simulink model "vehicle_motion_model_final_temp"  (R2021b)
settings: Solver=ode5  StartTime=0.0  StopTime=600  FixedStep=0.001  RelTol=1e-3
StopFcn:
  | % stop simulation callback function
  | figure(1);
  | out.x_gt.data = permute(out.x_gt.data,[3, 1, 2]);
  | plot3(out.x_gt.data(:, 1), out.x_gt.data(:, 2), -out.x_gt.data(:, 3), 'Color', 'r', 'LineWidth', 1.5);
  | legend('Истинная траектория')
  | xlabel('X, \itм');
  | ylabel('Y, \itм');
  | zlabel('Z, \itм');
  | figure(2);
  | plot3(out.x.data(:, 1), out.x.data(:, 2), -out.x.data(:, 3), 'Color', 'b', 'LineWidth', 1.5);
  | hold on;
  | xlabel('X, \itм');
  | ylabel('Y, \itм');
  | zlabel('Z, \itм');
  | % legend('pos')
  | hold on;
  | plot3(out.x_gt.data(:, 1), out.x_gt.data(:, 2), -out.x_gt.data(:, 3), 'Color', 'r', 'LineWidth', 1.5);
  | hold on;
  | legend('Рассчитанная траектория', 'Истинная траектория')
  | % errors
  | figure(3);
  | yyaxis left;
  | plot(out.hor_err_fus.time, out.hor_err_fus.data, 'Color', 'b', 'LineWidth', 1.5);
  | xlabel('время, \itс');
  | ylabel('Горизонтальная ошибка, \itм');
  | hold on;
  | yyaxis right;
  | plot(out.ver_err_fus.time, out.ver_err_fus.data, 'Color', 'r', 'LineWidth', 1.5);
  | ylabel('Вертикальная ошибка, \itм');
  | legend('Горизонтальная позиционная ошибка', 'Вертикальная позиционная ошибка');
  | grid on;
  | figure(4);
  | yyaxis left;
  | plot(out.hor_err_ins.time, out.hor_err_ins.data, '-', 'Color', 'b', 'LineWidth', 1.5);
  | xlabel('время, \itс');
  | ylabel('Горизонтальная ошибка, \itм');
  | hold on;
  | yyaxis right;
  | plot(out.ver_err_ins.time, out.ver_err_ins.data, '-', 'Color', 'r', 'LineWidth', 1.5);
  | ylabel('Вертикальная ошибка, \itм');
  | legend('Горизонтальная позиционная ошибка', 'Вертикальная позиционная ошибка');
  | grid on;
model workspace (MAT data in the model file):
  AxlIxx = 62.3745166667
  AxlM = 160
  Cps = 2
  CzWhlAxl = 557955.087061
  DCT_Param : object (value not decoded)
  Downshift_Speeds = [9.5625 12.9375 16.3125 19.6875 23.0625 26.4375 29.8125 33.1875 36.5625 39.9375 43.3125 46.6875 ... (28 elements, 4x7)]
  F0zWhlAxl = 16132.2380068
  HTCH : object (value not decoded)
  Hmax = 0.25
  KzWhlAxl = 58428920.0848
  NCyl = 6
  Pedal_Positions = [0.1 0.4 0.5 0.9]
  Pstd = 101325
  Q = [1  0  0; 0  1  0; 0  0  1]
  Rair = 287
  SUS : object (value not decoded)
  TRA : object (value not decoded)
  Trans : object (value not decoded)
  Tstd = 293.15
  Upshift_Speeds = [12.9375 16.3125 19.6875 33 26.4375 29.8125 33.1875 52.5 39.9375 43.3125 46.6875 77.25 ... (28 elements, 4x7)]
  VEH : object (value not decoded)
  Vd = 0.00346
  WH : Mass (value not decoded)
  dt3D = 0.05
  f_air = [0 0 0 0 0 0 0 0 0 0 0 0 ... (256 elements, 16x16)]
  f_co = [0 0 0 0 0 0 0 0 0 0 0 0 ... (256 elements, 16x16)]
  f_co2 = [0 0 0 0 0 0 0 0 0 0 0 0 ... (256 elements, 16x16)]
  f_eff = [352.135682859 352.135682859 320.724378192 303.655312657 295.930136708 291.240087194 291.240271258 291.240312459 291.240275452 291.240198499 291.240100781 291.240018769 ... (256 elements, 16x16)]
  f_fuel = [0 0 0 0 0 0 0 0 0 0 0 0 ... (256 elements, 16x16)]
  f_hc = [0 0 0 0 0 0 0 0 0 0 0 0 ... (256 elements, 16x16)]
  f_nox = [0 0 0 0 0 0 0 0 0 0 0 0 ... (256 elements, 16x16)]
  f_pm = [0 0 0 0 0 0 0 0 0 0 0 0 ... (256 elements, 16x16)]
  f_susp_axl_bp = [1 2]
  f_susp_dz_bp = [-0.325022776267 -0.315022776267 -0.305022776267 -0.205022776267 -0.105022776267 -0.00502277626717 0.0949772237328 0.194977223733 0.204977223733 0.214977223733]
  f_susp_dzdot_bp = [-3 -0.3 -0.2 -0.1 0 0.1 0.2 0.3 3]
  f_susp_fmz = [-144070.391448 -93629.24037 -75929.1118915 -20630.5828179 -15385.48216 -10140.3815021 -4895.28084414 349.819813785 -31916.3973792 18437.6709544 -83996.1993354 -33555.0482577 ... (43920 elements, 10x9x61x2x4)]
  f_susp_geom = [0 0 0 0 0 0 0 0 0 0 0 0 ... (3660 elements, 10x61x2x3)]
  f_susp_strgdelta_bp = [-0.523598775598 -0.506145483078 -0.488692190558 -0.471238898038 -0.453785605519 -0.436332312999 -0.418879020479 -0.401425727959 -0.383972435439 -0.366519142919 -0.349065850399 -0.331612557879 ... (61 elements, 1x61)]
  f_tbrake = [0 76.8593923996 105.140482948 131.533638111 157.926793274 176.658631717 176.65727296 176.656856686 176.656879077 176.657093756 176.657404516 176.65772406 ... (256 elements, 16x16)]
  f_tbrake_n_bpt = [0 649.519052838 912.419621844 1175.32019085 1438.22075986 1701.12132886 1964.02189787 2226.92246687 2489.82303588 2752.72360489 3015.62417389 3278.5247429 ... (16 elements, 1x16)]
  f_tbrake_t_bpt = [0 34.6410161514 61.0341713143 87.4273264773 113.82048164 140.213636803 166.606791966 192.999947129 219.393102292 245.786257455 272.179412618 298.572567781 ... (16 elements, 1x16)]
  f_texh = [766.752464599 766.752464599 786.17542386 801.679939032 884.591982581 910.574397722 910.571871054 910.570774534 910.570601632 910.570821151 910.571247242 910.571639815 ... (256 elements, 16x16)]
  f_twc_eff_co = [0.17 0.25 0.45 0.99 0.99 0.99 0.99]
  f_twc_eff_hc = [0.21 0.375 0.75 0.98 0.98 0.98 0.98]
  f_twc_eff_lam = [0.909090909 0.944055944 0.979020979 1 1.013986014 1.048951049 1.083916084]
  f_twc_eff_nox = [0.98 0.98 0.98 0.97 0.05 0.02 0]
  h = 0.134
symbols that are objects in the model workspace (value not decoded): VEH
libraries: aerolibcommonsys x8, sharedtransform x8, sharedutil x7, autolibsharedcommon x7, autolibutils x4, vehdynlibtirecommon x3, dspstat3 x2, mspsensorlib x1, aerolibnav x1, shared6dof x1, autolibshared x1, vehdynlibsuspension x1
(part 3 of 9)

== system vehicle_motion_model_final_temp/BINS/Three-axis Inertial Measurement Unit4 ==
  A_b : Inport  Unit=m/s^2  PortDimensions=3
  w : Inport  Port=2  Unit=rad/s  PortDimensions=3
  w_dot : Inport  Port=3  Unit=rad/s^2  PortDimensions=3
  CG : Inport  Port=4  Unit=m  PortDimensions=3
  g : Inport  Port=5  Unit=m/s^2  PortDimensions=3
  Acceleration Conversion : Subsystem
  Disallow CGS : UnitConfiguration  UnitSystemsStr=English,SI,SI (extended)  AllowAllUnitSystems=off
  Three-axis Accelerometer : Subsystem  AncestorBlock=aerolibnav/Three-axis Accelerometer  mask(Three-axis Accelerometer){units=Metric (MKS), acc=imu, gtype=on, dtype_a=off, w_a=w_a, z_a=z_a, a_sf_cc=a_sf_cc, a_bias=a_bias, a_Ts=i_Ts, a_rand=on, a_seeds=i_seeds(1:3), a_pow=i_pow(1:3), a_sat=a_sat}
      mask prompts: units "aeroblks:aeroblknav:blockThreeaxisAccelerometerParamUnits"; acc "aeroblks:aeroblknav:blockThreeaxisAccelerometerParamAccelerometerlocation"; gtype "aeroblks:aeroblknav:blockThreeaxisAccelerometerParamSubtractgravity"; dtype_a "aeroblks:aeroblknav:blockThreeaxisAccelerometerParamSecondorderdynamics"; w_a "aeroblks:aeroblknav:blockThreeaxisAccelerometerParamNaturalfrequencyradsec"; z_a "aeroblks:aeroblknav:blockThreeaxisAccelerometerParamDampingratio"; a_sf_cc "aeroblks:aeroblknav:blockThreeaxisAccelerometerParamScalefactorsandcrosscoupling"; a_bias "aeroblks:aeroblknav:blockThreeaxisAccelerometerParamMeasurementbias"; a_Ts "aeroblks:aeroblknav:blockThreeaxisAccelerometerParamUpdateratesec"; a_rand "aeroblks:aeroblknav:blockThreeaxisAccelerometerParamNoiseon"; a_seeds "aeroblks:aeroblknav:blockThreeaxisAccelerometerParamNoiseseeds"; a_pow "aeroblks:aeroblknav:blockThreeaxisAccelerometerParamNoisepower"; a_sat "aeroblks:aeroblknav:blockThreeaxisAccelerometerParamLowerandupperoutputlimits"
      mask help: aeroblks:aeroblknav:blockThreeaxisAccelerometerDesc
      mask init:
      | par = a_Ts;
      | block = gcb;
      | ports=aeroicon('aeroblkaccel','icon',par);
      | a_satl = a_sat(1:3);
      | a_sath = a_sat(4:6);
      mask Help: eval('asbhelp');
      mask TypeOptions units: aeroblks:aeroblknav:blockThreeaxisAccelerometerParamComboMetricMKS | aeroblks:aeroblknav:blockThreeaxisAccelerometerParamComboEnglish
      mask Callback gtype: aeroicon('aeroblkaccel')
      mask Callback dtype_a: aeroicon('aeroblkaccel')
      mask Callback a_rand: aeroicon('aeroblkaccel')
      mask DialogControl ParameterTabVar0 Prompt: Main
      mask DialogControl units Prompt: Units:
      mask DialogControl acc Prompt: Accelerometer location:
      mask DialogControl gtype Prompt: Subtract gravity:
      mask DialogControl dtype_a Prompt: Second-order dynamics
      mask DialogControl w_a Prompt: Natural frequency (rad/sec):
      mask DialogControl z_a Prompt: Damping ratio:
      mask DialogControl a_sf_cc Prompt: Scale factors and cross-coupling:
      mask DialogControl a_bias Prompt: Measurement bias:
      mask DialogControl a_Ts Prompt: Update rate (sec):
      mask DialogControl ParameterTabVar01 Prompt: Noise
      mask DialogControl a_rand Prompt: Noise on
      mask DialogControl a_seeds Prompt: Noise seeds:
      mask DialogControl a_pow Prompt: Noise power:
      mask DialogControl a_sat Prompt: Lower and upper output limits:
      mask Display:
      | port_label(ports(1).type,ports(1).port,ports(1).txt,'texmode','on');
      | port_label(ports(2).type,ports(2).port,ports(2).txt,'texmode','on');
      | port_label(ports(3).type,ports(3).port,ports(3).txt,'texmode','on');
      | port_label(ports(4).type,ports(4).port,ports(4).txt,'texmode','on');
      | port_label(ports(5).type,ports(5).port,ports(5).txt,'texmode','on');
      | port_label(ports(6).type,ports(6).port,ports(6).txt,'texmode','on');
  Three-axis Gyroscope : Subsystem  AncestorBlock=aerolibnav/Three-axis Gyroscope  mask(Three-axis Gyroscope){dtype_g=off, w_g=w_g, z_g=z_g, g_sf_cc=g_sf_cc, g_bias=g_bias, g_sen=g_sens, g_Ts=i_Ts, g_rand=on, g_seeds=i_seeds(4:6), g_pow=i_pow(4:6), g_sat=g_sat}
      mask prompts: dtype_g "aeroblks:aeroblknav:blockThreeaxisGyroscopeParamSecondorderdynamics"; w_g "aeroblks:aeroblknav:blockThreeaxisGyroscopeParamNaturalfrequencyradsec"; z_g "aeroblks:aeroblknav:blockThreeaxisGyroscopeParamDampingratio"; g_sf_cc "aeroblks:aeroblknav:blockThreeaxisGyroscopeParamScalefactorsandcrosscoupling"; g_bias "aeroblks:aeroblknav:blockThreeaxisGyroscopeParamMeasurementbias"; g_sen "aeroblks:aeroblknav:blockThreeaxisGyroscopeParamGsensitivebias"; g_Ts "aeroblks:aeroblknav:blockThreeaxisGyroscopeParamUpdateratesec"; g_rand "aeroblks:aeroblknav:blockThreeaxisGyroscopeParamNoiseon"; g_seeds "aeroblks:aeroblknav:blockThreeaxisGyroscopeParamNoiseseeds"; g_pow "aeroblks:aeroblknav:blockThreeaxisGyroscopeParamNoisepower"; g_sat "aeroblks:aeroblknav:blockThreeaxisGyroscopeParamLowerandupperoutputlimits"
      mask help: aeroblks:aeroblknav:blockThreeaxisGyroscopeDesc
      mask init:
      | par = g_Ts;
      | block = gcb;
      | g_satl = g_sat(1:3);
      | g_sath = g_sat(4:6);
      | ports=aeroicon('aeroblkgyro','icon',par);
      mask Help: eval('asbhelp');
      mask Callback dtype_g: aeroicon('aeroblkgyro');
      mask Callback g_rand: aeroicon('aeroblkgyro');
      mask DialogControl ParameterTabVar0 Prompt: Main
      mask DialogControl dtype_g Prompt: Second-order dynamics
      mask DialogControl w_g Prompt: Natural frequency (rad/sec):
      mask DialogControl z_g Prompt: Damping ratio:
      mask DialogControl g_sf_cc Prompt: Scale factors and cross-coupling:
      mask DialogControl g_bias Prompt: Measurement bias:
      mask DialogControl g_sen Prompt: G-sensitive bias:
      mask DialogControl g_Ts Prompt: Update rate (sec):
      mask DialogControl ParameterTabVar01 Prompt: Noise
      mask DialogControl g_rand Prompt: Noise on
      mask DialogControl g_seeds Prompt: Noise seeds:
      mask DialogControl g_pow Prompt: Noise power:
      mask DialogControl g_sat Prompt: Lower and upper output limits:
      mask Display:
      | port_label(ports(1).type,ports(1).port,ports(1).txt,'texmode','on');
      | port_label(ports(2).type,ports(2).port,ports(2).txt,'texmode','on');
      | port_label(ports(3).type,ports(3).port,ports(3).txt,'texmode','on');
  A_meas : Outport  Unit=m/s^2  VectorParamsAs1DForOutWhenUnconnected=off
  w_meas : Outport  Port=2  Unit=rad/s  VectorParamsAs1DForOutWhenUnconnected=off
  wires:
  g/1 -> Three-axis Accelerometer/5(g)
  Acceleration Conversion/1(inherit) -> Three-axis Gyroscope/2(G's)
  w_dot/1 -> Three-axis Accelerometer/3(pdot qdot rdot)
  CG/1 -> Three-axis Accelerometer/4(CG)
  w/1 -> Three-axis Accelerometer/2(p q r), Three-axis Gyroscope/1(p q r)
  A_b/1 -> Three-axis Accelerometer/1(Ab), Acceleration Conversion/1(acceleration)
  Three-axis Gyroscope/1((p q r)_meas) -> w_meas/1
  Three-axis Accelerometer/1(Ameas) -> A_meas/1

== system vehicle_motion_model_final_temp/BINS kinematics Euler/Subsystem ==
  True : Inport
  BINS : Inport  Port=2
  Scope1 : Scope  NumInputPorts=3
  Sum2 : Sum  Inputs=+-|
  wires:
  True/1 -> Sum2/1, Scope1/1
  BINS/1 -> Scope1/2, Sum2/2
  Sum2/1 -> Scope1/3

== system vehicle_motion_model_final_temp/BINS kinematics Euler/Subsystem1 ==
  True : Inport
  BINS : Inport  Port=2
  Scope1 : Scope  NumInputPorts=3
  Sum2 : Sum  Inputs=+-|
  wires:
  True/1 -> Sum2/1, Scope1/1
  BINS/1 -> Scope1/2, Sum2/2
  Sum2/1 -> Scope1/3

== system vehicle_motion_model_final_temp/Calc errors/Subsystem ==
  <Disp> : Inport
  <CalcPos> : Inport  Port=2
  Abs : Abs
  Selector : Selector  InputPortWidth=3  IndexOptions=Index vector (dialog)  Indices=[1]  OutputSizes=1
  Selector1 : Selector  InputPortWidth=3  IndexOptions=Index vector (dialog)  Indices=[1]  OutputSizes=1
  Selector2 : Selector  InputPortWidth=3  IndexOptions=Index vector (dialog)  Indices=[2]  OutputSizes=1
  Selector3 : Selector  InputPortWidth=3  IndexOptions=Index vector (dialog)  Indices=[2]  OutputSizes=1
  Selector4 : Selector  InputPortWidth=3  IndexOptions=Index vector (dialog)  Indices=[3]  OutputSizes=1
  Selector5 : Selector  InputPortWidth=3  IndexOptions=Index vector (dialog)  Indices=[3]  OutputSizes=1
  Square : Math  Operator=square  SaturateOnIntegerOverflow=on
  Square Root : Sqrt  SaturateOnIntegerOverflow=on
  Square1 : Math  Operator=square  SaturateOnIntegerOverflow=on
  Sum : Sum  Inputs=+-
  Sum1 : Sum  Inputs=-+
  Sum4 : Sum  Inputs=+-
  Sum5 : Sum
  HorError : Outport
  VertError : Outport  Port=2
  wires:
  Square Root/1 -> HorError/1
  Selector/1 -> Sum/1
  Square1/1 -> Sum5/2
  Sum4/1 -> Square1/1
  Sum/1 -> Square/1
  Selector3/1 -> Sum4/2
  Selector1/1 -> Sum/2
  Selector2/1 -> Sum4/1
  Square/1 -> Sum5/1
  Sum5/1 -> Square Root/1
  <CalcPos>/1 -> Selector1/1, Selector4/1, Selector3/1
  Selector5/1 -> Sum1/2
  <Disp>/1 -> Selector5/1, Selector2/1, Selector/1
  Selector4/1 -> Sum1/1
  Sum1/1 -> Abs/1
  Abs/1 -> VertError/1

== system vehicle_motion_model_final_temp/Calc errors1/Subsystem1 ==
  <Disp> : Inport
  <CalcPos> : Inport  Port=2
  Abs : Abs
  Selector : Selector  InputPortWidth=3  IndexOptions=Index vector (dialog)  Indices=[1]  OutputSizes=1
  Selector1 : Selector  InputPortWidth=3  IndexOptions=Index vector (dialog)  Indices=[1]  OutputSizes=1
  Selector2 : Selector  InputPortWidth=3  IndexOptions=Index vector (dialog)  Indices=[2]  OutputSizes=1
  Selector3 : Selector  InputPortWidth=3  IndexOptions=Index vector (dialog)  Indices=[2]  OutputSizes=1
  Selector4 : Selector  InputPortWidth=3  IndexOptions=Index vector (dialog)  Indices=[3]  OutputSizes=1
  Selector5 : Selector  InputPortWidth=3  IndexOptions=Index vector (dialog)  Indices=[3]  OutputSizes=1
  Square : Math  Operator=square  SaturateOnIntegerOverflow=on
  Square Root : Sqrt  SaturateOnIntegerOverflow=on
  Square1 : Math  Operator=square  SaturateOnIntegerOverflow=on
  Sum : Sum  Inputs=+-
  Sum1 : Sum  Inputs=-+
  Sum4 : Sum  Inputs=+-
  Sum5 : Sum
  HorError : Outport
  VertError : Outport  Port=2
  wires:
  Square Root/1 -> HorError/1
  Selector/1 -> Sum/1
  Square1/1 -> Sum5/2
  Sum4/1 -> Square1/1
  Sum/1 -> Square/1
  Selector3/1 -> Sum4/2
  Selector1/1 -> Sum/2
  Selector2/1 -> Sum4/1
  Square/1 -> Sum5/1
  Sum5/1 -> Square Root/1
  <CalcPos>/1 -> Selector1/1, Selector4/1, Selector3/1
  Selector5/1 -> Sum1/2
  <Disp>/1 -> Selector5/1, Selector2/1, Selector/1
  Selector4/1 -> Sum1/1
  Sum1/1 -> Abs/1
  Abs/1 -> VertError/1

== system vehicle_motion_model_final_temp/Calc errors2/Subsystem ==
  <Disp> : Inport
  <CalcPos> : Inport  Port=2
  Abs : Abs
  Selector : Selector  InputPortWidth=3  IndexOptions=Index vector (dialog)  Indices=[1]  OutputSizes=1
  Selector1 : Selector  InputPortWidth=3  IndexOptions=Index vector (dialog)  Indices=[1]  OutputSizes=1
  Selector2 : Selector  InputPortWidth=3  IndexOptions=Index vector (dialog)  Indices=[2]  OutputSizes=1
  Selector3 : Selector  InputPortWidth=3  IndexOptions=Index vector (dialog)  Indices=[2]  OutputSizes=1
  Selector4 : Selector  InputPortWidth=3  IndexOptions=Index vector (dialog)  Indices=[3]  OutputSizes=1
  Selector5 : Selector  InputPortWidth=3  IndexOptions=Index vector (dialog)  Indices=[3]  OutputSizes=1
  Square : Math  Operator=square  SaturateOnIntegerOverflow=on
  Square Root : Sqrt  SaturateOnIntegerOverflow=on
  Square1 : Math  Operator=square  SaturateOnIntegerOverflow=on
  Sum : Sum  Inputs=+-
  Sum1 : Sum  Inputs=-+
  Sum4 : Sum  Inputs=+-
  Sum5 : Sum
  HorError : Outport
  VertError : Outport  Port=2
  wires:
  Square Root/1 -> HorError/1
  Selector/1 -> Sum/1
  Square1/1 -> Sum5/2
  Sum4/1 -> Square1/1
  Sum/1 -> Square/1
  Selector3/1 -> Sum4/2
  Selector1/1 -> Sum/2
  Selector2/1 -> Sum4/1
  Square/1 -> Sum5/1
  Sum5/1 -> Square Root/1
  <CalcPos>/1 -> Selector1/1, Selector4/1, Selector3/1
  Selector5/1 -> Sum1/2
  <Disp>/1 -> Selector5/1, Selector2/1, Selector/1
  Selector4/1 -> Sum1/1
  Sum1/1 -> Abs/1
  Abs/1 -> VertError/1

== system vehicle_motion_model_final_temp/Calc errors3/Subsystem ==
  <Disp> : Inport
  <CalcPos> : Inport  Port=2
  Abs : Abs
  Selector : Selector  InputPortWidth=3  IndexOptions=Index vector (dialog)  Indices=[1]  OutputSizes=1
  Selector1 : Selector  InputPortWidth=3  IndexOptions=Index vector (dialog)  Indices=[1]  OutputSizes=1
  Selector2 : Selector  InputPortWidth=3  IndexOptions=Index vector (dialog)  Indices=[2]  OutputSizes=1
  Selector3 : Selector  InputPortWidth=3  IndexOptions=Index vector (dialog)  Indices=[2]  OutputSizes=1
  Selector4 : Selector  InputPortWidth=3  IndexOptions=Index vector (dialog)  Indices=[3]  OutputSizes=1
  Selector5 : Selector  InputPortWidth=3  IndexOptions=Index vector (dialog)  Indices=[3]  OutputSizes=1
  Square : Math  Operator=square  SaturateOnIntegerOverflow=on
  Square Root : Sqrt  SaturateOnIntegerOverflow=on
  Square1 : Math  Operator=square  SaturateOnIntegerOverflow=on
  Sum : Sum  Inputs=+-
  Sum1 : Sum  Inputs=-+
  Sum4 : Sum  Inputs=+-
  Sum5 : Sum
  HorError : Outport
  VertError : Outport  Port=2
  wires:
  Square Root/1 -> HorError/1
  Selector/1 -> Sum/1
  Square1/1 -> Sum5/2
  Sum4/1 -> Square1/1
  Sum/1 -> Square/1
  Selector3/1 -> Sum4/2
  Selector1/1 -> Sum/2
  Selector2/1 -> Sum4/1
  Square/1 -> Sum5/1
  Sum5/1 -> Square Root/1
  <CalcPos>/1 -> Selector1/1, Selector4/1, Selector3/1
  Selector5/1 -> Sum1/2
  <Disp>/1 -> Selector5/1, Selector2/1, Selector/1
  Selector4/1 -> Sum1/1
  Sum1/1 -> Abs/1
  Abs/1 -> VertError/1

== system vehicle_motion_model_final_temp/Prediction step (BINS)/Initial State ==
  Bus Selector : BusSelector  OutputSignals=Disp,Vel,Ang
  Constant10 : Constant  Value=[0;0;0]
  Mux3 : Mux  Inputs=6
  Rotation Angles to Quaternions2 : sharedtransform/Rotation Angles to Quaternions  rotationOrder=ZYX  aMode=aMode
      settings: SourceProductBaseCode=AE,PW,DR,MT,UV,VE
  Selector2 : Selector  InputPortWidth=3  IndexOptions=Index vector (dialog)  Indices=[3 2 1]  OutputSizes=1
  Out1 : Outport
  wires:
  Mux3/1 -> Out1/1
  [g] -> Mux3/6
  Bus Selector/3 -> Selector2/1  "<Ang>"
  Bus Selector/1 -> Mux3/1  "<Disp>"
  Rotation Angles to Quaternions2/1 -> Mux3/3
  Bus Selector/2 -> Mux3/2  "<Vel>"
  Constant10/1 -> Mux3/5, Mux3/4
  Selector2/1 -> Rotation Angles to Quaternions2/1
  [InertFrmCg] -> Bus Selector/1

== system vehicle_motion_model_final_temp/Prediction step (BINS)/Subsystem4 ==
  Clock1 : Clock
  Memory : Memory
  Scope : Scope
  Sum : Sum  Inputs=+-
  dT : Outport  VectorParamsAs1DForOutWhenUnconnected=off
  wires:
  Clock1/1 -> Sum/1, Memory/1
  Memory/1 -> Sum/2
  Sum/1 -> Scope/1, dT/1

== system vehicle_motion_model_final_temp/Sensor fusion/Initial State ==
  Bus Selector : BusSelector  OutputSignals=Disp,Vel,Ang
  Constant10 : Constant  Value=[0;0;0]
  Mux3 : Mux  Inputs=6
  Rotation Angles to Quaternions2 : sharedtransform/Rotation Angles to Quaternions  rotationOrder=ZYX  aMode=aMode
      settings: SourceProductBaseCode=AE,PW,DR,MT,UV,VE
  Selector2 : Selector  InputPortWidth=3  IndexOptions=Index vector (dialog)  Indices=[3 2 1]  OutputSizes=1
  Out1 : Outport
  wires:
  Mux3/1 -> Out1/1
  [g] -> Mux3/6
  Bus Selector/3 -> Selector2/1  "<Ang>"
  Bus Selector/1 -> Mux3/1  "<Disp>"
  Rotation Angles to Quaternions2/1 -> Mux3/3
  Bus Selector/2 -> Mux3/2  "<Vel>"
  Constant10/1 -> Mux3/5, Mux3/4
  Selector2/1 -> Rotation Angles to Quaternions2/1
  [InertFrmCg] -> Bus Selector/1

== system vehicle_motion_model_final_temp/Sensor fusion/Subsystem4 ==
  Clock1 : Clock
  Memory : Memory
  Scope : Scope
  Sum : Sum  Inputs=+-
  dT : Outport  VectorParamsAs1DForOutWhenUnconnected=off
  wires:
  Clock1/1 -> Sum/1, Memory/1
  Memory/1 -> Sum/2
  Sum/1 -> Scope/1, dT/1

== system vehicle_motion_model_final_temp/Two-Axle Vehicle/Vehicle Body ==
  Suspension : Inport
  Vehicle Body 6DOF : Subsystem  VariantControl=1
  Vehicle : Outport

== system vehicle_motion_model_final_temp/Two-Axle Vehicle/Vehicle Suspension ==
  Steering : Inport
  Wheels : Inport  Port=2
  Vehicle : Inport  Port=3
  Bus Creator1 : BusCreator  Inputs=5
  Bus Creator2 : BusCreator  Inputs=2
  Bus Creator3 : BusCreator  Inputs=2
  Bus Creator4 : BusCreator  Inputs=6
  Bus Selector : BusSelector  OutputSignals=z,Re,zdot,Fx,Fy,M
  Bus Selector1 : BusSelector  OutputSignals=P,V
  Selector1 : Selector  NumberOfDimensions=2  InputPortWidth=3  IndexOptions=Index vector (dialog),Select all  Indices=1,1  OutputSizes=1,1
  Selector2 : Selector  NumberOfDimensions=2  InputPortWidth=3  IndexOptions=Index vector (dialog),Select all  Indices=2,1  OutputSizes=1,1
  Solid Axle Suspension - Coil Spring : vehdynlibsuspension/Solid Axle Suspension - Coil Spring  NumAxl=2  NumTracksByAxl=[2 2]  StrgEnByAxl=[1 1]  TrackNumVec="[1  2  1  2]"  AxleNumVec="[1  1  2  2]"  SuspTypesByAxle="[1  1]"  SuspImage=suspsacoil.png  AxlIxx=450  AxlM=500  TrackCoords="[zeros(1,4);VEH.TrackWidth*[1 -1  1 -1]/2;zeros(1,4)]"  SuspCoords="[zeros(1,4);VEH.TrackWidth*[1 -1  1 -1]/2;zeros(1,4)]"  KzWhlAxl=KzWhlAxl  F0zWhlAxl=F0zWhlAxl  CzWhlAxl=CzWhlAxl  IdealSuspEn=on  IdealSuspAxles="[1  2]"  Kz=VEH.Kz  F0z=VEH.F0z  Cz=VEH.Cz  Hmax=Hmax  Toe=0  RollStrgSlp=0  ToeStrgSlp=0  Caster=0  CasterHslp=0  CasterStrgSlp=0  Camber=0  CamberHslp=0  CamberStrgSlp=0  StrgHgtSlp=0.1432  MappedSuspEn=off  MappedSuspAxles="[1  2]"  f_susp_axl_bp=[1 2]  f_susp_dz_bp=[-0.15 -0.14 -0.13 -0.12 -0.11 -0.10 -0.09 -0.08 -0.07 -0.06 -0.05 -0.04 -0.03 -0.02 -0.01 0.00 0.01 0.02 0.03 0.04 0.05 0.06 0.07 0.08 0.09 0.10 0.11 0.12 0.13 0.14 0.15]  f_susp_dzdot_bp=[-0.15 -0.14 -0.13 -0.12 -0.11 -0.10 -0.09 -0.08 -0.07 -0.06 -0.05 -0.04 -0.03 -0.02 -0.01 0.00 0.01 0.02 0.03 0.04 0.05 0.06 0.07 0.08 0.09 0.10 0.11 0.12 0.13 0.14 0.15]  f_susp_fmz=zeros(31,31,61,2,4)  f_susp_geom=zeros(31,61,2,3)  f_susp_strgdelta_bp=[-30,-29,-28,-27,-26,-25,-24,-23,-22,-21,-20,-19,-18,-17,-16,-15,-14,-13,-12,-11,-10,-9,-8,-7,-6,-5,-4,-3,-2,-1,0,1,2,3,4,5,6,7,8,9,10,11,12,13,14,15,16,17,18,19,20,21,22,23,24,25,26,27,28,29,30]
      settings: SourceProductBaseCode=VE
  Steer Rate Adapter : Subsystem
  Steering Adapter : Subsystem
  Terminator : Terminator
  Terminator6 : Terminator
  Vehicle Adapter : Subsystem
  Wheel  Adapter : Subsystem
  Z Force Splice : Subsystem  Variant=on  VariantControlMode=label  LabelModeActiveChoice=1
  Suspension : Outport
  wires:
  Wheel  Adapter/6(Re) -> Bus Creator4/6
  Bus Selector1/1 -> Solid Axle Suspension - Coil Spring/7  "<P>"
  Bus Selector/6 -> Solid Axle Suspension - Coil Spring/6  "<M>"
  Bus Selector/1 -> Solid Axle Suspension - Coil Spring/1  "<z>"
  Bus Selector/5 -> Solid Axle Suspension - Coil Spring/5  "<Fy>"
  Wheel  Adapter/1(WhlFx) -> Bus Creator4/1  "Fx"
  Bus Selector/4 -> Solid Axle Suspension - Coil Spring/4  "<Fx>"
  Wheel  Adapter/4(zdot) -> Bus Creator4/4
  Wheel  Adapter/2(WhlFy) -> Bus Creator4/2  "Fy"
  Solid Axle Suspension - Coil Spring/1 -> Terminator6/1
  Vehicle Adapter/1(VehSusp) -> Bus Selector1/1
  Bus Creator4/1 -> Bus Selector/1
  Bus Selector1/2 -> Solid Axle Suspension - Coil Spring/8  "<V>"
  Steering/1 -> Steering Adapter/1(Steer)
  Bus Selector/3 -> Solid Axle Suspension - Coil Spring/3  "<zdot>"
  Wheel  Adapter/3(z) -> Bus Creator4/3
  Wheel  Adapter/5(M) -> Bus Creator4/5
  Bus Selector/2 -> Solid Axle Suspension - Coil Spring/2  "<Re>"
  Vehicle Adapter/2(VehVbody) -> Selector1/1, Selector2/1
  Wheels/1 -> Wheel  Adapter/1(Wheels)
  Steering Adapter/1(StrgAng) -> Solid Axle Suspension - Coil Spring/9
  Vehicle/1 -> Vehicle Adapter/1(Veh), Z Force Splice/3(Vehicle), Steer Rate Adapter/1(Veh)
  Bus Creator3/1 -> Suspension/1
  Selector2/1 -> Bus Creator1/3  "ydot"
  Solid Axle Suspension - Coil Spring/4 -> Z Force Splice/2(WhlFIn)
  Bus Creator2/1 -> Bus Creator3/1  "Veh"
  Solid Axle Suspension - Coil Spring/3 -> Bus Creator2/2  "M"
  Selector1/1 -> Bus Creator1/2  "xdot"
  Solid Axle Suspension - Coil Spring/6 -> Bus Creator1/4  "Ang"
  Solid Axle Suspension - Coil Spring/2 -> Z Force Splice/1(VehFIn)
  Bus Creator1/1 -> Bus Creator3/2  "Whl"
  Steer Rate Adapter/1(AngVel) -> Bus Creator1/5
  Z Force Splice/1(VehF) -> Bus Creator2/1  "F"
  Z Force Splice/2(WhlF) -> Bus Creator1/1  "F"
  Solid Axle Suspension - Coil Spring/5 -> Terminator/1

== system vehicle_motion_model_final_temp/Two-Axle Vehicle/Wheels and Tires ==
  Suspension : Inport
  Axle Torque : Inport  Port=2
  Brake Press : Inport  Port=3  Unit=Pa
  Ground Input : Inport  Port=4
  Friction : Inport  Port=5
  Bus Selector1 : BusSelector  OutputSignals=Whl.Ang,Whl.F,Whl.AngVel,Whl.xdot,Whl.ydot
  Constant3 : Constant  Value=zeros(4,1)
  Cont LPF : autolibutils/Cont LPF  wc=100*2*pi  aMode=2
      settings: SourceProductBaseCode=PW,DR,MT,UV,VE
  Cont LPF1 : autolibutils/Cont LPF  wc=100*2*pi  aMode=2
      settings: SourceProductBaseCode=PW,DR,MT,UV,VE
  Manual Switch6 : ManualSwitch
  Matrix Concatenate : Concatenate  NumInputs=3  Mode=Multidimensional array
  Reshape1 : Reshape
  Reshape2 : Reshape
  Reshape3 : Reshape  OutputDimensionality=Column vector (2-D)
  Reshape4 : Reshape
  Selector : Selector  NumberOfDimensions=2  InputPortWidth=3  IndexOptions=Index vector (dialog),Select all  Indices=[3],1  OutputSizes=1,1
  Selector1 : Selector  NumberOfDimensions=2  InputPortWidth=1  IndexOptions=Index vector (dialog),Select all  Indices=[3],1  OutputSizes=1,1
  Selector2 : Selector  NumberOfDimensions=2  InputPortWidth=3  IndexOptions=Index vector (dialog),Select all  Indices=3,1  OutputSizes=1,1
  Selector3 : Selector  NumberOfDimensions=2  InputPortWidth=3  IndexOptions=Index vector (dialog),Select all  Indices=1,1  OutputSizes=1,1
  Terminator{,1,3..5} (5 alike) : Terminator
  Wheels and Tires : Subsystem  VariantControl=0
  z forces per tire : Subsystem
  Wheels : Outport  VectorParamsAs1DForOutWhenUnconnected=off
  wires:
  Wheels and Tires/1(WhlAng) -> Wheels/1  "Wheels"
  Bus Selector1/2 -> Selector/1  "<F>"
  Wheels and Tires/2(FrntAxlF) -> Terminator/1
  Wheels and Tires/3(RearAxlF) -> Terminator1/1
  Wheels and Tires/4(Omega) -> Terminator3/1
  Wheels and Tires/5(Mz) -> Terminator4/1
  Selector1/1 -> Reshape1/1
  Matrix Concatenate/1 -> Wheels and Tires/7(VehVel)
  Axle Torque/1 -> Wheels and Tires/3(AxleTrq)
  Selector2/1 -> Wheels and Tires/1(WheelAng)  "Wheel Angles"
  Constant3/1 -> Manual Switch6/1
  Manual Switch6/1 -> Wheels and Tires/2(CamberAng)  "Camber Angles"
  Selector/1 -> Reshape2/1
  z forces per tire/1(FzTire) -> Wheels and Tires/5(Fz)
  Ground Input/1 -> Wheels and Tires/8(Ground Level)
  Wheels and Tires/7(SuspWhlVz) -> Matrix Concatenate/3  "zdot"
  Bus Selector1/1 -> Cont LPF1/1  "<Ang>"
  Selector3/1 -> Reshape3/1  "Camber Angles"
  Suspension/1 -> Bus Selector1/1
  Bus Selector1/4 -> Matrix Concatenate/1  "<xdot>"
  Bus Selector1/5 -> Matrix Concatenate/2  "<ydot>"
  Wheels and Tires/6(SuspWhlPz) -> Terminator5/1  "z"
  Reshape2/1 -> Cont LPF/1
  Bus Selector1/3 -> Selector1/1  "<AngVel>"
  Reshape1/1 -> Wheels and Tires/6(r)
  Brake Press/1 -> Wheels and Tires/4(BrkPrs)
  Friction/1 -> Wheels and Tires/9(Friction)
  Cont LPF1/1 -> Selector3/1, Selector2/1
  Reshape3/1 -> Reshape4/1  "Camber Angles"
  Reshape4/1 -> Manual Switch6/2  "Camber Angles"
  Cont LPF/1 -> z forces per tire/1(FzIn)

== system vehicle_motion_model_final_temp/BINS/Three-axis Inertial Measurement Unit2/Acceleration Conversion ==
  acceleration : Inport  Unit=m/s^2
  Unit Conversion : UnitConversion
  inherit : Outport  VectorParamsAs1DForOutWhenUnconnected=off
  wires:
  Unit Conversion/1 -> inherit/1
  acceleration/1 -> Unit Conversion/1

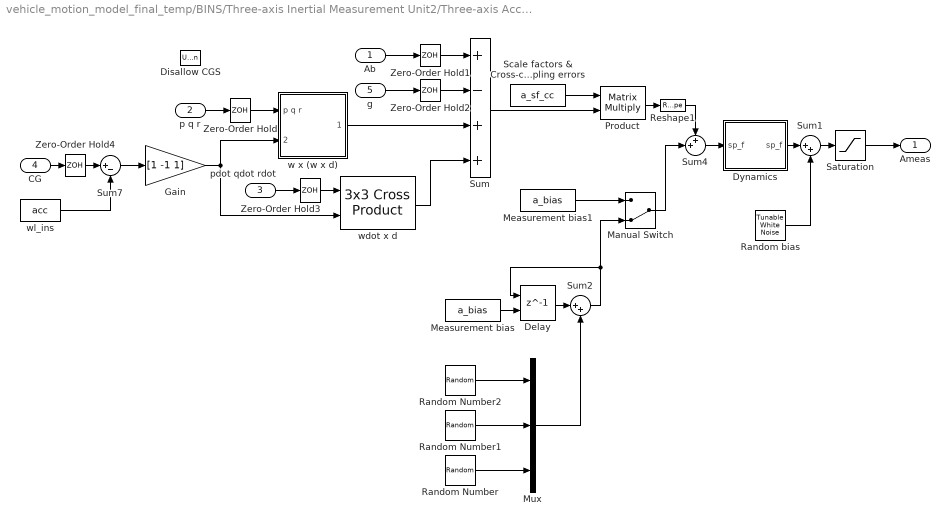
== system vehicle_motion_model_final_temp/BINS/Three-axis Inertial Measurement Unit2/Three-axis Accelerometer ==
  Ab : Inport  Unit=m/s^2  PortDimensions=3
  p q r : Inport  Port=2  Unit=rad/s  PortDimensions=3
  pdot qdot rdot : Inport  Port=3  Unit=rad/s^2  PortDimensions=3
  CG : Inport  Port=4  Unit=m  PortDimensions=3
  g : Inport  Port=5  Unit=m/s^2  PortDimensions=3
  Delay : Delay  DelayLength=1  InitialConditionSource=Input port  InitialCondition=0
      settings: InputPortMap=u0,p4
  Disallow CGS : UnitConfiguration  UnitSystemsStr=English,SI,SI (extended)  AllowAllUnitSystems=off
  Dynamics : Subsystem
  Gain : Gain  Gain=[1 -1 1]  SaturateOnIntegerOverflow=on  OutDataTypeStr=Inherit: Same as input  ParamDataTypeStr=Inherit: Same as input
  Manual Switch : ManualSwitch  CurrentSetting=0
  Measurement bias : Constant  Value=a_bias
  Measurement bias1 : Constant  Value=a_bias
  Mux : Mux  Inputs=3
  Product : Product  Multiplication=Matrix(*)  SaturateOnIntegerOverflow=on  OutDataTypeStr=Inherit: Same as first input
  Random Number : RandomNumber  Variance=2e-8  Seed=42347548753  SampleTime=a_Ts
  Random Number1 : RandomNumber  Variance=2e-8  Seed=95834573489579834  SampleTime=a_Ts
  Random Number2 : RandomNumber  Variance=2e-8  Seed=974128941341343  SampleTime=a_Ts
  Random bias : aerolibcommonsys/Tunable White Noise  pwr=a_pow  Ts=a_Ts  seed=a_seeds
      settings: SourceProductBaseCode=AE
  Reshape1 : Reshape
  Saturation : Saturate  UpperLimit=a_sath  LowerLimit=a_satl
  Scale factors & Cross-coupling errors : Constant  Value=a_sf_cc
  Sum : Sum  Inputs=+-++  SaturateOnIntegerOverflow=on
  Sum1 : Sum  Inputs=|++  SaturateOnIntegerOverflow=on
  Sum2 : Sum  Inputs=|++  SaturateOnIntegerOverflow=on
  Sum4 : Sum  Inputs=++|  SaturateOnIntegerOverflow=on
  Sum7 : Sum  Inputs=|+-  SaturateOnIntegerOverflow=on
  Zero-Order Hold{,1..4} (5 alike) : ZeroOrderHold  SampleTime=a_Ts
  w x (w x d) : Subsystem
  wdot x d : sharedutil/3x3 Cross Product  aMode=aMode
      settings: SourceProductBaseCode=AE,PW,DR,MT,UV,VE
  wl_ins : Constant  Value=acc
  Ameas : Outport  Unit=m/s^2  PortDimensions=3  VectorParamsAs1DForOutWhenUnconnected=off
  wires:
  Saturation/1 -> Ameas/1
  Random bias/1 -> Sum1/2
  Scale factors & Cross-coupling errors/1 -> Product/1
  wdot x d/1 -> Sum/4
  Sum/1 -> Product/2
  p q r/1 -> Zero-Order Hold/1
  pdot qdot rdot/1 -> Zero-Order Hold3/1
  CG/1 -> Zero-Order Hold4/1
  Product/1 -> Reshape1/1
  Reshape1/1 -> Sum4/1
  Ab/1 -> Zero-Order Hold1/1
  w x (w x d)/1(w x ( w x d)) -> Sum/3
  Sum1/1 -> Saturation/1
  Sum4/1 -> Dynamics/1(sp_f)
  Dynamics/1("sp_f ") -> Sum1/1
  Sum7/1 -> Gain/1
  wl_ins/1 -> Sum7/2
  Gain/1 -> w x (w x d)/2(distance), wdot x d/2
  g/1 -> Zero-Order Hold2/1
  Zero-Order Hold1/1 -> Sum/1
  Zero-Order Hold2/1 -> Sum/2
  Zero-Order Hold/1 -> w x (w x d)/1("p q r ")
  Zero-Order Hold3/1 -> wdot x d/1
  Zero-Order Hold4/1 -> Sum7/1
  Measurement bias/1 -> Delay/2
  Delay/1 -> Sum2/1
  Random Number2/1 -> Mux/1
  Random Number1/1 -> Mux/2
  Random Number/1 -> Mux/3
  Mux/1 -> Sum2/2
  Measurement bias1/1 -> Manual Switch/1
  Sum2/1 -> Delay/1, Manual Switch/2
  Manual Switch/1 -> Sum4/2

== system vehicle_motion_model_final_temp/BINS/Three-axis Inertial Measurement Unit2/Three-axis Gyroscope ==
  p q r : Inport  Unit=rad/s  PortDimensions=3
  G's : Inport  Port=2  Unit=gn  PortDimensions=3
  Delay : Delay  DelayLength=1  InitialConditionSource=Input port  InitialCondition=0
      settings: InputPortMap=u0,p4
  Disallow CGS : UnitConfiguration  UnitSystemsStr=English,SI,SI (extended)  AllowAllUnitSystems=off
  Dynamics : Subsystem
  Manual Switch : ManualSwitch  CurrentSetting=0
  Measurement bias : Constant  Value=g_bias
  Measurement bias1 : Constant  Value=g_bias
  Mux : Mux  Inputs=3
  Product : Product  Multiplication=Matrix(*)  SaturateOnIntegerOverflow=on  OutDataTypeStr=Inherit: Same as first input
  Product1 : Product  SaturateOnIntegerOverflow=on  OutDataTypeStr=Inherit: Same as first input
  Random Number : RandomNumber  Variance=2e-14  Seed=32454353467  SampleTime=g_Ts
  Random Number1 : RandomNumber  Variance=2e-14  Seed=34523523  SampleTime=g_Ts
  Random Number2 : RandomNumber  Variance=2e-14  Seed=325326557  SampleTime=g_Ts
  Random bias : aerolibcommonsys/Tunable White Noise  pwr=g_pow  Ts=g_Ts  seed=g_seeds
      settings: SourceProductBaseCode=AE
  Saturation : Saturate  UpperLimit=g_sath  LowerLimit=g_satl
  "Scale factors & Cross-coupling errors " : Constant  Value=g_sf_cc
  Sum1 : Sum  Inputs=|++  SaturateOnIntegerOverflow=on
  Sum2 : Sum  Inputs=|++  SaturateOnIntegerOverflow=on
  Sum4 : Sum  Inputs=+++  SaturateOnIntegerOverflow=on
  Zero-Order Hold : ZeroOrderHold  SampleTime=g_Ts
  Zero-Order Hold1 : ZeroOrderHold  SampleTime=g_Ts
  g-sensitive bias : Constant  Value=g_sen
  (p q r)_meas : Outport  Unit=rad/s  PortDimensions=3  VectorParamsAs1DForOutWhenUnconnected=off
  wires:
  Product/1 -> Sum4/1
  Sum4/1 -> Dynamics/1(p q r)
  "Scale factors & Cross-coupling errors "/1 -> Product/1
  Random bias/1 -> Sum1/2
  Saturation/1 -> (p q r)_meas/1
  p q r/1 -> Zero-Order Hold/1
  g-sensitive bias/1 -> Product1/2
  Sum1/1 -> Saturation/1
  G's/1 -> Zero-Order Hold1/1
  Dynamics/1("p q r ") -> Sum1/1
  Product1/1 -> Sum4/3
  Zero-Order Hold/1 -> Product/2
  Zero-Order Hold1/1 -> Product1/1
  Delay/1 -> Sum2/1
  Measurement bias/1 -> Delay/2
  Mux/1 -> Sum2/2
  Random Number/1 -> Mux/1
  Manual Switch/1 -> Sum4/2
  Measurement bias1/1 -> Manual Switch/1
  Random Number1/1 -> Mux/2
  Random Number2/1 -> Mux/3
  Sum2/1 -> Delay/1, Manual Switch/2

== system vehicle_motion_model_final_temp/BINS/Three-axis Inertial Measurement Unit4/Acceleration Conversion ==
  acceleration : Inport  Unit=m/s^2
  Unit Conversion : UnitConversion
  inherit : Outport  VectorParamsAs1DForOutWhenUnconnected=off
  wires:
  Unit Conversion/1 -> inherit/1
  acceleration/1 -> Unit Conversion/1

== system vehicle_motion_model_final_temp/BINS/Three-axis Inertial Measurement Unit4/Three-axis Accelerometer ==
  Ab : Inport  Unit=m/s^2  PortDimensions=3
  p q r : Inport  Port=2  Unit=rad/s  PortDimensions=3
  pdot qdot rdot : Inport  Port=3  Unit=rad/s^2  PortDimensions=3
  CG : Inport  Port=4  Unit=m  PortDimensions=3
  g : Inport  Port=5  Unit=m/s^2  PortDimensions=3
  Delay : Delay  DelayLength=1  InitialConditionSource=Input port  InitialCondition=0
      settings: InputPortMap=u0,p4
  Disallow CGS : UnitConfiguration  UnitSystemsStr=English,SI,SI (extended)  AllowAllUnitSystems=off
  Dynamics : Subsystem
  Gain : Gain  Gain=[1 -1 1]  SaturateOnIntegerOverflow=on  OutDataTypeStr=Inherit: Same as input  ParamDataTypeStr=Inherit: Same as input
  Manual Switch : ManualSwitch  CurrentSetting=0
  Measurement bias : Constant  Value=a_bias
  Measurement bias1 : Constant  Value=a_bias
  Mux : Mux  Inputs=3
  Product : Product  Multiplication=Matrix(*)  SaturateOnIntegerOverflow=on  OutDataTypeStr=Inherit: Same as first input
  Random Number : RandomNumber  Variance=24e-6  Seed=42347548753  SampleTime=a_Ts
  Random Number1 : RandomNumber  Variance=24e-6  Seed=95834573489579834  SampleTime=a_Ts
  Random Number2 : RandomNumber  Variance=24e-6  Seed=974128941341343  SampleTime=a_Ts
  Random bias : aerolibcommonsys/Tunable White Noise  pwr=a_pow  Ts=a_Ts  seed=a_seeds
      settings: SourceProductBaseCode=AE
  Reshape1 : Reshape
  Saturation : Saturate  UpperLimit=a_sath  LowerLimit=a_satl
  Scale factors & Cross-coupling errors : Constant  Value=a_sf_cc
  Sum : Sum  Inputs=+-++  SaturateOnIntegerOverflow=on
  Sum1 : Sum  Inputs=|++  SaturateOnIntegerOverflow=on
  Sum2 : Sum  Inputs=|++  SaturateOnIntegerOverflow=on
  Sum4 : Sum  Inputs=++|  SaturateOnIntegerOverflow=on
  Sum7 : Sum  Inputs=|+-  SaturateOnIntegerOverflow=on
  Zero-Order Hold{,1..4} (5 alike) : ZeroOrderHold  SampleTime=a_Ts
  w x (w x d) : Subsystem
  wdot x d : sharedutil/3x3 Cross Product  aMode=aMode
      settings: SourceProductBaseCode=AE,PW,DR,MT,UV,VE
  wl_ins : Constant  Value=acc
  Ameas : Outport  Unit=m/s^2  PortDimensions=3  VectorParamsAs1DForOutWhenUnconnected=off
  wires:
  Saturation/1 -> Ameas/1
  Random bias/1 -> Sum1/2
  Scale factors & Cross-coupling errors/1 -> Product/1
  wdot x d/1 -> Sum/4
  Sum/1 -> Product/2
  p q r/1 -> Zero-Order Hold/1
  pdot qdot rdot/1 -> Zero-Order Hold3/1
  CG/1 -> Zero-Order Hold4/1
  Product/1 -> Reshape1/1
  Reshape1/1 -> Sum4/1
  Ab/1 -> Zero-Order Hold1/1
  w x (w x d)/1(w x ( w x d)) -> Sum/3
  Sum1/1 -> Saturation/1
  Sum4/1 -> Dynamics/1(sp_f)
  Dynamics/1("sp_f ") -> Sum1/1
  Sum7/1 -> Gain/1
  wl_ins/1 -> Sum7/2
  Gain/1 -> w x (w x d)/2(distance), wdot x d/2
  g/1 -> Zero-Order Hold2/1
  Zero-Order Hold1/1 -> Sum/1
  Zero-Order Hold2/1 -> Sum/2
  Zero-Order Hold/1 -> w x (w x d)/1("p q r ")
  Zero-Order Hold3/1 -> wdot x d/1
  Zero-Order Hold4/1 -> Sum7/1
  Measurement bias/1 -> Delay/2
  Delay/1 -> Sum2/1
  Random Number2/1 -> Mux/1
  Random Number1/1 -> Mux/2
  Random Number/1 -> Mux/3
  Mux/1 -> Sum2/2
  Measurement bias1/1 -> Manual Switch/1
  Sum2/1 -> Delay/1, Manual Switch/2
  Manual Switch/1 -> Sum4/2

== system vehicle_motion_model_final_temp/BINS/Three-axis Inertial Measurement Unit4/Three-axis Gyroscope ==
  p q r : Inport  Unit=rad/s  PortDimensions=3
  G's : Inport  Port=2  Unit=gn  PortDimensions=3
  Delay : Delay  DelayLength=1  InitialConditionSource=Input port  InitialCondition=0
      settings: InputPortMap=u0,p4
  Disallow CGS : UnitConfiguration  UnitSystemsStr=English,SI,SI (extended)  AllowAllUnitSystems=off
  Dynamics : Subsystem
  Manual Switch : ManualSwitch  CurrentSetting=0
  Measurement bias : Constant  Value=g_bias
  Measurement bias1 : Constant  Value=g_bias
  Mux : Mux  Inputs=3
  Product : Product  Multiplication=Matrix(*)  SaturateOnIntegerOverflow=on  OutDataTypeStr=Inherit: Same as first input
  Product1 : Product  SaturateOnIntegerOverflow=on  OutDataTypeStr=Inherit: Same as first input
  Random Number : RandomNumber  Variance=1.2e-10  Seed=32454353467  SampleTime=g_Ts
  Random Number1 : RandomNumber  Variance=1.2e-10  Seed=34523523  SampleTime=g_Ts
  Random Number2 : RandomNumber  Variance=1.2e-10  Seed=325326557  SampleTime=g_Ts
  Random bias : aerolibcommonsys/Tunable White Noise  pwr=g_pow  Ts=g_Ts  seed=g_seeds
      settings: SourceProductBaseCode=AE
  Saturation : Saturate  UpperLimit=g_sath  LowerLimit=g_satl
  "Scale factors & Cross-coupling errors " : Constant  Value=g_sf_cc
  Sum1 : Sum  Inputs=|++  SaturateOnIntegerOverflow=on
  Sum2 : Sum  Inputs=|++  SaturateOnIntegerOverflow=on
  Sum4 : Sum  Inputs=+++  SaturateOnIntegerOverflow=on
  Zero-Order Hold : ZeroOrderHold  SampleTime=g_Ts
  Zero-Order Hold1 : ZeroOrderHold  SampleTime=g_Ts
  g-sensitive bias : Constant  Value=g_sen
  (p q r)_meas : Outport  Unit=rad/s  PortDimensions=3  VectorParamsAs1DForOutWhenUnconnected=off
  wires:
  Product/1 -> Sum4/1
  Sum4/1 -> Dynamics/1(p q r)
  "Scale factors & Cross-coupling errors "/1 -> Product/1
  Random bias/1 -> Sum1/2
  Saturation/1 -> (p q r)_meas/1
  p q r/1 -> Zero-Order Hold/1
  g-sensitive bias/1 -> Product1/2
  Sum1/1 -> Saturation/1
  G's/1 -> Zero-Order Hold1/1
  Dynamics/1("p q r ") -> Sum1/1
  Product1/1 -> Sum4/3
  Zero-Order Hold/1 -> Product/2
  Zero-Order Hold1/1 -> Product1/1
  Delay/1 -> Sum2/1
  Measurement bias/1 -> Delay/2
  Mux/1 -> Sum2/2
  Random Number/1 -> Mux/1
  Manual Switch/1 -> Sum4/2
  Measurement bias1/1 -> Manual Switch/1
  Random Number1/1 -> Mux/2
  Random Number2/1 -> Mux/3
  Sum2/1 -> Delay/1, Manual Switch/2
